simulink model "test"  (R2015a)
settings: Solver=ode45  StartTime=0.0  StopTime=100  RelTol=1e-3
undefined symbols (not defined in the file): L, R
libraries: simulink x2
settings Model: Creator=dell  LastModifiedBy=dell

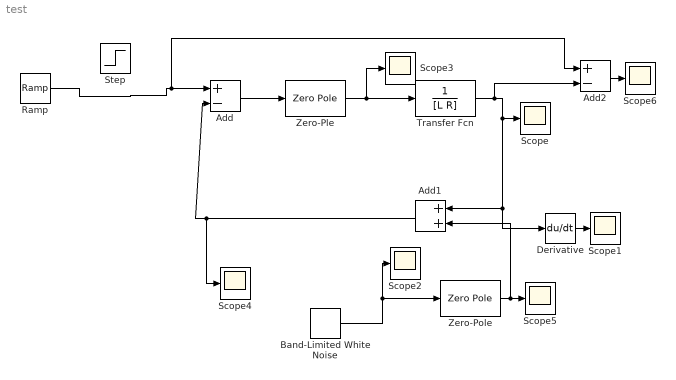
== system test ==
  Add : Sum  Inputs=+-
  Add1 : Sum
  Add2 : Sum  Inputs=+-
  Band-Limited White Noise : simulink/Sources/Band-Limited White Noise  Cov=[1]  Ts=1/200  seed=[23341]
  Derivative : Derivative
  Ramp : simulink/Sources/Ramp  slope=0.2  start=0  X0=0
  Scope{,1..6} (7 alike) : Scope
      Scope settings: YMin=-2.5  YMax=17.5  MaxDataPoints=500000
      Scope1 settings: YMin=0.63  YMax=0.73  MaxDataPoints=500000
      Scope2 settings: YMin=0.63  YMax=0.73  SaveName=ScopeData2  MaxDataPoints=500000
      Scope3 settings: TimeRange=10  YMin=0.63  YMax=0.73  SaveName=ScopeData3  MaxDataPoints=500000
      Scope4 settings: YMin=0.63  YMax=0.73  SaveName=ScopeData4  MaxDataPoints=500000
      Scope5 settings: YMin=0.63  YMax=0.73  SaveName=ScopeData5  MaxDataPoints=500000
      Scope6 settings: YMin=-0.01  YMax=0.01  SaveName=ScopeData6  MaxDataPoints=500000
  Step : Step  After=100  SampleTime=0
  Transfer Fcn : TransferFcn  Denominator=[L R]
  Zero-Ple : ZeroPole  Zeros=[-0.18]  Poles=[0,0]  Gain=[1.1379]
  Zero-Pole : ZeroPole  Zeros=[0]  Poles=[-5 -100,-150]  Gain=[150]
  wires:
  Transfer Fcn/1 -> Add2/2, Add1/1, Derivative/1, Scope/1
  Add1/1 -> Scope4/1, Add/2
  Derivative/1 -> Scope1/1
  Band-Limited White Noise/1 -> Zero-Pole/1, Scope2/1
  Zero-Ple/1 -> Scope3/1, Transfer Fcn/1
  Add/1 -> Zero-Ple/1
  Zero-Pole/1 -> Add1/2, Scope5/1
  Ramp/1 -> Add2/1, Add/1
  Add2/1 -> Scope6/1
